simulink model "Waehrungsmodelle"  (R2014a)
settings: Solver=ode1  StartTime=0.0  StopTime=100  FixedStep=1  MaxStep=1  MinStep=1  RelTol=1e-3
(part 7 of 18)

== matlab function Waehrungsmodelle/Vollgeld Währungssystem/Banken/MATLAB Function ==
  data: EinlagenAenderungHaushalte input; KreditbedarfHaushalte input; KreditbedarfUnternehmen input; KreditbedarfHaushalteAusland input; KreditbedarfUnternehmenAusland input; KreditbedarfStaat input; Steuersatz input; Leitzins input; Mindestreservesatz input; MaximaleNotenbankGeldmenge input; KontoHaushalteOut output; KrediteHaushalteOut output; KrediteUnternehmenOut output; KrediteStaatOut output; KreditvergabeHaushalte output; KreditvergabeUnternehmen output; KreditvergabeStaat output; KreditrueckzahlungHaushalte output; KreditrueckzahlungUnternehmen output; KreditrueckzahlungStaat output; BankgewinnNachSteuern output; BankenSteuern output; BankKontostand output; Bankenzinssatz output; KrediteUnternehmenAuslandOut output; KreditrueckzahlungUnternehmenAusland output; KreditvergabeUnternehmenAusland output; KrediteHaushalteAuslandOut output; KreditrueckzahlungHaushalteAusland output; KreditvergabeHaushalteAusland output
function [KontoHaushalteOut, KrediteHaushalteOut, KrediteUnternehmenOut, KrediteStaatOut, ... 
            KreditvergabeHaushalte, KreditvergabeUnternehmen, KreditvergabeStaat, ...
            KreditrueckzahlungHaushalte, KreditrueckzahlungUnternehmen, KreditrueckzahlungStaat, ...
            BankgewinnNachSteuern, BankenSteuern, BankKontostand, Bankenzinssatz, ...
            KrediteUnternehmenAuslandOut, KreditrueckzahlungUnternehmenAusland, KreditvergabeUnternehmenAusland, ...
            KrediteHaushalteAuslandOut, KreditrueckzahlungHaushalteAusland, KreditvergabeHaushalteAusland] = ...
    Banken(EinlagenAenderungHaushalte, KreditbedarfHaushalte, KreditbedarfUnternehmen, ...
            KreditbedarfHaushalteAusland, KreditbedarfUnternehmenAusland, KreditbedarfStaat, ...
            Steuersatz, Leitzins, Mindestreservesatz, MaximaleNotenbankGeldmenge)
% Submodell Banken zur Berechnung der Geld-Prozesse zwischen 
% Banken und Haushalten

% ANMERKUNG:
% Warum gibt es auf der einen Seite Kredite und Guthaben der Haushalte?
% Der überwigende Teil der Geldes MUSS den Haushalten gehören, da diese
% die Unternehmen und Banken besitzen. Ich vermute, dass es in einen
% demokratischen Staat nicht möglich ist, dass der Staat mehr Geld als 
% die Bevölkerung besitzt.
% Die ungleiche Geldverteilung ist dafür verantwortlich, dass die Haushalte
% auf der einen Seite Spareinlagen und Kredite haben. Ohne Spareinlagen wäre
% es aktuell nicht möglich Kredite überhaupt zu vergeben.

% Der Zinsspread ist die Prozentuale-Differenz der Zinsweitergabe bei
% Krediten und Anlagen
persistent Zinsspread;

% interner Zinssatz
persistent InternerZinssatz;

% aktuelle Kredithöhe der Unternehmen
persistent KrediteUnternehmen;

% aktuelle Kredithöhe des Staats
persistent KrediteStaat;

% aktuelle Kredithöhe der Haushalte
persistent KrediteHaushalte;

% aktuelle Kredithöhe der Unternehmen im Ausland
persistent KrediteUnternehmenAusland;

% aktuelle Kredithöhe der Haushalte im Ausland
persistent KrediteHaushalteAusland;

% aktueller Kontostand der Haushalte
persistent KontoHaushalte;

% Rückzahlungsdauer des Kredits
persistent Kreditrueckzahlungsdauer;

% Vermnögen der Bank aus den Gewinnen
persistent KontoBank;

    % Zinsspread 1%
    if isempty(Zinsspread)
       Zinsspread = 0.01;
    end 
    
    % interner Zinssatz auf den Leitzins festlegen
    if isempty(InternerZinssatz)
       InternerZinssatz = Leitzins;
    end     
    
    % Rückzahlungsdauer 15 Zeiteinheiten
    if isempty(Kreditrueckzahlungsdauer)
       Kreditrueckzahlungsdauer = 15;
    end     
   
    if isempty(KontoBank)
       KontoBank = 400;
    end   
    if isempty(KontoHaushalte)
       KontoHaushalte = 0;
    end   
    if isempty(KrediteHaushalte)
       KrediteHaushalte = 200;
    end     
    if isempty(KrediteUnternehmen)
       KrediteUnternehmen = 200;
    end 
    if isempty(KrediteStaat)
       KrediteStaat = 200;
    end     
    if isempty(KrediteUnternehmenAusland)
       KrediteUnternehmenAusland = 200;
    end     
    if isempty(KrediteHaushalteAusland)
       KrediteHaushalteAusland = 200;
    end   
    
    % Zinsspread an das Guthaben der Bank anpassen
    if KontoBank < 0
        Zinsspread = Zinsspread + 0.01;
    elseif KontoBank > 1000
        Zinsspread = max(Zinsspread - 0.01, 0.01);
    end
    
    % Habenzinsen berechnen
    HabenZinsen = KontoHaushalte * (InternerZinssatz - Zinsspread);
    KontoHaushalte = KontoHaushalte + HabenZinsen;
    
    % Ein- / Auszahlung
    KontoHaushalte = KontoHaushalte + EinlagenAenderungHaushalte;    
      
    % Maximale Kreditvergabe anhand des Mindestreservesatzes und der 
    % Spareinlagen der Haushalte
    MaximaleKreditvergabe = KontoHaushalte * (1 / Mindestreservesatz); 

    % Maximale Geldmenge, welche von der Notenbank zur Verfügung gestellt wird
    % Prüfung anhand der Maximalen Kreditvergabe, da Guthaben = Kredit    
    MaximaleKreditvergabe = max(MaximaleNotenbankGeldmenge, MaximaleKreditvergabe);
    
    Gesamtkredit = KrediteHaushalte + KrediteUnternehmen + KrediteStaat;
    MaximaleKreditvergabe = MaximaleKreditvergabe - Gesamtkredit;

    % Wenn genug Geld auf dem Konto ist, so wird ein prozenualer Anteil mit
    % dem neuen Kreditbedarf verrechnet ==> 10 %    
    if KontoHaushalte > KreditbedarfHaushalte && KreditbedarfHaushalte > 0
       AusgleichbarerGeldBedarf = KreditbedarfHaushalte * 0.1;
       KontoHaushalte = KontoHaushalte - AusgleichbarerGeldBedarf;
       KreditbedarfHaushalte = KreditbedarfHaushalte - AusgleichbarerGeldBedarf;
    end         

    % Kreditberechnung für Haushalte      
    [KrediteHaushalte, KreditvergabeHaushalte, KreditrueckzahlungHaushalte, ...
                        SollZinsenHaushalte, MaximaleKreditvergabe] = ...
        Kreditberechnung(KrediteHaushalte, KreditbedarfHaushalte, MaximaleKreditvergabe, ...
                        InternerZinssatz, Zinsspread, Kreditrueckzahlungsdauer);                    
    
    % Kreditberechnung für Staat   
    [KrediteStaat, KreditvergabeStaat, KreditrueckzahlungStaat, SollZinsenStaat, ...
                        MaximaleKreditvergabe] = ...
        Kreditberechnung(KrediteStaat, KreditbedarfStaat, MaximaleKreditvergabe, ...
                        InternerZinssatz, Zinsspread, Kreditrueckzahlungsdauer);                    

    % Kreditberechnung für Unternehmen   
    [KrediteUnternehmen, KreditvergabeUnternehmen, KreditrueckzahlungUnternehmen, ...
                        SollZinsenUnternehmen, MaximaleKreditvergabe] = ...
        Kreditberechnung(KrediteUnternehmen, KreditbedarfUnternehmen, MaximaleKreditvergabe, ...
                        InternerZinssatz, Zinsspread, Kreditrueckzahlungsdauer);

    % Kreditberechnung für Haushalte im Ausland
    [KrediteHaushalteAusland, KreditvergabeHaushalteAusland, KreditrueckzahlungHaushalteAusland, ...
                        SollZinsenHaushalteAusland, MaximaleKreditvergabe] = ...
        Kreditberechnung(KrediteHaushalteAusland, KreditbedarfHaushalteAusland, MaximaleKreditvergabe, ...
                        InternerZinssatz, Zinsspread, Kreditrueckzahlungsdauer);                                        

    % Kreditberechnung für Unternehmen im Ausland
    [KrediteUnternehmenAusland, KreditvergabeUnternehmenAusland, KreditrueckzahlungUnternehmenAusland, ...
                        SollZinsenUnternehmenAusland, MaximaleKreditvergabe] = ...
        Kreditberechnung(KrediteUnternehmenAusland, KreditbedarfUnternehmenAusland, MaximaleKreditvergabe, ...
                        InternerZinssatz, Zinsspread, Kreditrueckzahlungsdauer);                    
                    
    % Berechnung der Notenbankkredite
    NotenbankKredite = (KrediteHaushalte + KrediteUnternehmen + KrediteStaat + ...
                    KrediteHaushalteAusland + KrediteUnternehmenAusland) - (KontoBank + KontoHaushalte);
    NotenbankKredite = max(NotenbankKredite, 0);
    NotenbankZinsen = NotenbankKredite * Leitzins;
    KontoBank = KontoBank - NotenbankZinsen;   
    
    % Gewinnberechnung der Bank
    SollZinsen = SollZinsenHaushalte + SollZinsenStaat + SollZinsenUnternehmen ...
                + SollZinsenHaushalteAusland + SollZinsenUnternehmenAusland;
    Bankgewinn = SollZinsen - HabenZinsen;
    
    % Steuerberechnung der Bank
    BankenSteuern = max(Bankgewinn * Steuersatz, 0);
    BankgewinnNachSteuern = Bankgewinn - BankenSteuern;
    
    % Kontostand der Bank berechnen
    KontoBank = KontoBank + Bankgewinn - BankenSteuern;
    
    % Zinssätze anpassen (Zinsänderung anpassen y = -0.00005x + 0.0025;
    Zinsaenderung = -0.00005 * BankgewinnNachSteuern + 0.001;
    Zinsaenderung = min(0.01, max(Zinsaenderung, -0.01));
    InternerZinssatz = InternerZinssatz + Zinsaenderung;
    
    if InternerZinssatz > 1
       InternerZinssatz = 0.1; 
    end
    
    KrediteStaatOut = KrediteStaat;
    KrediteUnternehmenOut = KrediteUnternehmen;
    KrediteHaushalteOut = KrediteHaushalte;
    KrediteUnternehmenAuslandOut = KrediteUnternehmenAusland;
    KrediteHaushalteAuslandOut = KrediteHaushalteAusland;    
    KontoHaushalteOut = KontoHaushalte;    
    BankKontostand = KontoBank;
    Bankenzinssatz = InternerZinssatz;

== matlab function Waehrungsmodelle/Währungssystem3/Umwelt/Umwelt ==
  data: Ressourcenbedarf input; AbgebauteRessourcen output; VorhandeneRessourcenOut output; Umweltqualitaet output
function [AbgebauteRessourcen, VorhandeneRessourcenOut, Umweltqualitaet] = Umwelt(Ressourcenbedarf)
%# Submodell zum Prozessablauf der Umwelt und der Ressourcen


% Vorhandene Ressourcen
persistent VorhandeneRessourcen;

% Initiale Ressourcen
InitialeRessourcen = 2500;
% Maximale Abbaurate
MaximaleAbbaurate = 0.1;
% Ressourcenregenerationsrate
Ressourcenregenerationsrate = 0.02;
    
% Vorhandene Ressourcen Initial
if isempty(VorhandeneRessourcen)
   VorhandeneRessourcen = InitialeRessourcen;
end

    % Berechnung der maximal abbaubaren Ressourcen
    MaximalAbbaubareRessourcen = VorhandeneRessourcen * MaximaleAbbaurate;
    
    % abgebaute Ressourcen
    AbgebauteRessourcen = min(MaximalAbbaubareRessourcen, Ressourcenbedarf);       
    VorhandeneRessourcen = VorhandeneRessourcen - AbgebauteRessourcen;
    
    % Ressourcen Regeneration
    VorhandeneRessourcen = VorhandeneRessourcen * (1  + Ressourcenregenerationsrate);    
    
    % Umweltqualitaet berechnen
    Umweltqualitaet = max(min(VorhandeneRessourcen / InitialeRessourcen, 1), 0);
        
    VorhandeneRessourcenOut = VorhandeneRessourcen;

== matlab function Waehrungsmodelle/Währungssystem3/Wechselkursberechnung/MATLAB Function ==
  data: GueterpreisAuslandInEigenwaehrung output; GueterpreisAusland input; Wechselkursfaktor output; GueterKonsumImInlandVomAusland input; GueterKonsumImAuslandVomInland input; GesamterGueterKonsumImAuslandVomInlandOut output; GesamterGueterKonsumImInlandVomAuslandOut output
function [GueterpreisAuslandInEigenwaehrung, Wechselkursfaktor, GesamterGueterKonsumImAuslandVomInlandOut, GesamterGueterKonsumImInlandVomAuslandOut] ...
        = Wechselkursberechnung(GueterpreisAusland, GueterKonsumImInlandVomAusland, GueterKonsumImAuslandVomInland)
%# Untermodul zur Berechnung eines realen Wechselkurses


% Aufsummierter Güterkonsum vom Ausland mit produzierten Gütern aus dem Inland
persistent GesamterGueterKonsumImAuslandVomInland;          
        
% Aufsummierter Güterkonsum vom Inland mit produzierten Gütern aus dem Ausland
persistent GesamterGueterKonsumImInlandVomAusland;    

% GesamterGueterKonsumImAuslandVomInland Initial
if isempty(GesamterGueterKonsumImAuslandVomInland)
   GesamterGueterKonsumImAuslandVomInland = 1;
end

% GueterKonsumImInlandVomAusland Initial
if isempty(GesamterGueterKonsumImInlandVomAusland)
   GesamterGueterKonsumImInlandVomAusland = 1;
end

GesamterGueterKonsumImAuslandVomInland = GesamterGueterKonsumImAuslandVomInland + GueterKonsumImAuslandVomInland;
GesamterGueterKonsumImInlandVomAusland = GesamterGueterKonsumImInlandVomAusland + GueterKonsumImInlandVomAusland;
   
% Berechnung eines realen Wechselkurses
Wechselkursfaktor =  GesamterGueterKonsumImInlandVomAusland / GesamterGueterKonsumImAuslandVomInland;

% Güterpreis der importierten Waren in Inländischer Währung
GueterpreisAuslandInEigenwaehrung = GueterpreisAusland * Wechselkursfaktor;

% Zustandswerte ausgeben
GesamterGueterKonsumImAuslandVomInlandOut = GesamterGueterKonsumImAuslandVomInland;
GesamterGueterKonsumImInlandVomAuslandOut = GesamterGueterKonsumImInlandVomAusland;

== matlab function Waehrungsmodelle/Gedecktes Währungssystem/Deckungsmaterialschöpfung/MATLAB Function ==
  data: NachfrageDeckungsmaterial input; RessourcenMengeDeckungsmaterial output; PreisDeckungsmaterialOut output; AngebotsMengeDeckungsmaterial output; Ressourcenabbaumenge output
function [RessourcenMengeDeckungsmaterial, PreisDeckungsmaterialOut, AngebotsMengeDeckungsmaterial, Ressourcenabbaumenge] = ...
    SchoepfungDeckungsmaterial(NachfrageDeckungsmaterial)
%# Submodul zur Berechnung der Notenbankprozesse

% Abbauzyklen
persistent Abbauzyklus;

% abgebauter Vorrat an dem Deckungsmaterial
persistent VorratDeckungsmaterial;

% Preis des Deckungsmaterial
persistent PreisDeckungsmaterial;

    % Anfänglicher Preis für das Deckungsmaterial
    InitPreisDeckungsmaterial = 10;

    if isempty(VorratDeckungsmaterial)
       VorratDeckungsmaterial = 100;
    end  
    if isempty(Abbauzyklus)
       Abbauzyklus = 1;
    end  
    if isempty(PreisDeckungsmaterial)
       PreisDeckungsmaterial = InitPreisDeckungsmaterial;
    end  
        
    Abbauzyklus = Abbauzyklus + 1;
        
    % Abbaumenge pro Zeiteinheit
    Ressourcenabbaumenge = 70 - 20 * (Abbauzyklus ^ 0.2);    
    VorratDeckungsmaterial = VorratDeckungsmaterial + Ressourcenabbaumenge;
    
    if VorratDeckungsmaterial < NachfrageDeckungsmaterial * 3
        PreisAenderungsfaktor = max(1, NachfrageDeckungsmaterial / Ressourcenabbaumenge);
    elseif VorratDeckungsmaterial > NachfrageDeckungsmaterial * 25
        PreisAenderungsfaktor = min(1, max(0.9, NachfrageDeckungsmaterial / Ressourcenabbaumenge));
    else
        PreisAenderungsfaktor =  min(1.2, NachfrageDeckungsmaterial / Ressourcenabbaumenge);
    end
    
    PreisDeckungsmaterial = PreisDeckungsmaterial * (2+PreisAenderungsfaktor) / 3;
    
    % Auf Grund der Deckung ist der Preis für das Deckungsmaterial niemals
    % unter dem ursprünglichen Geld. Auf Grund des Angebots und der
    % Nachfrage ist es dennoch möglich, dass der Preis schwankt
    if PreisDeckungsmaterial < InitPreisDeckungsmaterial
        PreisDeckungsmaterial = InitPreisDeckungsmaterial;
    end
    
    if VorratDeckungsmaterial > NachfrageDeckungsmaterial
        AngebotsMengeDeckungsmaterial = NachfrageDeckungsmaterial;
        
    else
        AngebotsMengeDeckungsmaterial = VorratDeckungsmaterial;
    end
    
    VorratDeckungsmaterial = VorratDeckungsmaterial - AngebotsMengeDeckungsmaterial;           
    RessourcenMengeDeckungsmaterial = VorratDeckungsmaterial;
    PreisDeckungsmaterialOut = PreisDeckungsmaterial;

== matlab function Waehrungsmodelle/Gedecktes Währungssystem/Umwelt/Umwelt ==
  data: Ressourcenbedarf input; AbgebauteRessourcen output; VorhandeneRessourcenOut output; Umweltqualitaet output
function [AbgebauteRessourcen, VorhandeneRessourcenOut, Umweltqualitaet] = Umwelt(Ressourcenbedarf)
%# Submodell zum Prozessablauf der Umwelt und der Ressourcen


% Vorhandene Ressourcen
persistent VorhandeneRessourcen;

% Initiale Ressourcen
InitialeRessourcen = 2500;
% Maximale Abbaurate
MaximaleAbbaurate = 0.1;
% Ressourcenregenerationsrate
Ressourcenregenerationsrate = 0.02;
    
% Vorhandene Ressourcen Initial
if isempty(VorhandeneRessourcen)
   VorhandeneRessourcen = InitialeRessourcen;
end

    % Berechnung der maximal abbaubaren Ressourcen
    MaximalAbbaubareRessourcen = VorhandeneRessourcen * MaximaleAbbaurate;
    
    % abgebaute Ressourcen
    AbgebauteRessourcen = min(MaximalAbbaubareRessourcen, Ressourcenbedarf);       
    VorhandeneRessourcen = VorhandeneRessourcen - AbgebauteRessourcen;
    
    % Ressourcen Regeneration
    VorhandeneRessourcen = VorhandeneRessourcen * (1  + Ressourcenregenerationsrate);    
    
    % Umweltqualitaet berechnen
    Umweltqualitaet = max(min(VorhandeneRessourcen / InitialeRessourcen, 1), 0);
        
    VorhandeneRessourcenOut = VorhandeneRessourcen;

== matlab function Waehrungsmodelle/Gedecktes Währungssystem/Unternehmen/MATLAB Function ==
  data: Inflation output; Rohstoffbedarf output; ArbeitsplaetzeUnternehmen output; GueterangebotInland output; ArbeitslohnOut output; Erwerbsfaehige input; BenoetigterArbeitsbedarfUnternehmen output; GueterpreisOut output; NeueKreditvergabeUnternehmen input; KreditrueckzahlungUnternehmen input; SteuernUnternehmen output; RessourcenAbgabeSteuer output; KreditbedarfInland output; Rohstoffe input; GueterkonsumInland input; GueterkonsumAusland input; RessourcenAbgabeSteuersatz input; KreditZinssatzInland input; KreditZinssatzAusland input; Steuersatz input; KreditbedarfAusland output; TechnischeVerbesserungRationalitaetOut output; TechnischeVerbesserungRessourcenOut output; Wirtschaftswachstum output; GueterangebotAusland output; NeueKreditvergabeUnternehmenAusland input; KreditrueckzahlungUnternehmenAusland input
function [Inflation, Rohstoffbedarf, ArbeitsplaetzeUnternehmen, GueterangebotInland, ...
            ArbeitslohnOut, BenoetigterArbeitsbedarfUnternehmen, GueterpreisOut, ...
            SteuernUnternehmen, RessourcenAbgabeSteuer, KreditbedarfInland, KreditbedarfAusland,  ...
            TechnischeVerbesserungRationalitaetOut, TechnischeVerbesserungRessourcenOut, ...
            Wirtschaftswachstum, GueterangebotAusland] = ...
   Unternehmen(Erwerbsfaehige, NeueKreditvergabeUnternehmen, KreditrueckzahlungUnternehmen, ...
            Rohstoffe, GueterkonsumInland, GueterkonsumAusland, RessourcenAbgabeSteuersatz, ...
            KreditZinssatzInland, KreditZinssatzAusland, Steuersatz, ...
            NeueKreditvergabeUnternehmenAusland, KreditrueckzahlungUnternehmenAusland)
        %# Submodul zur Berechnung der Prozessabläufe in Beziehung mit den Unternehmen

% Arbeitslohn
persistent Arbeitslohn;          
        
% Geldbestand
persistent Geldbestand;  
        
% Rohstoffbestand
persistent Rohstoffbestand;   
        
% produzierter Güterbestand
persistent Gueterbestand;   

% Preis zu dem das produzierte Gut verkauft wird
persistent Gueterpreis;  

% technische Effizienzverbesserung bzgl. der Rationalisierung der Arbeiter
persistent TechnischeVerbesserungRationalitaet;   

% technische Effizienzverbesserung bzgl. der Ressourcenverwendung
persistent TechnischeVerbesserungRessourcen;

% Letzte Anzahl an Mitarbeitern
persistent LetzteArbeitsplaetzeUnternehmen;

% Umsatz / Einnahmen
persistent Einnahmen;

% alte Inflation
persistent InflationAlt;

% Geldbestand Initial
if isempty(Geldbestand)
   Geldbestand = 50;
end
% Arbeitslohn Initial
if isempty(Arbeitslohn)
   Arbeitslohn = 3.5;
end
% Rohstoffbestand Initial
if isempty(Rohstoffbestand)
   Rohstoffbestand = 50;
end
% Güterbestand Initial
if isempty(Gueterbestand)
   Gueterbestand = 50;
end 
% Güterpreis Initial
if isempty(Gueterpreis)
   Gueterpreis = 3;
end 
% technische Effizienzverbesserung Rationalisierung Initial
if isempty(TechnischeVerbesserungRessourcen)
   TechnischeVerbesserungRessourcen = 1;
end
% technische Effizienzverbesserung Ressourcenverwendung Initial
if isempty(TechnischeVerbesserungRationalitaet)
   TechnischeVerbesserungRationalitaet = 1;
end
% Umsatz / Einnahmen Initial
if isempty(Einnahmen)
   Einnahmen = 0;
end
if isempty(InflationAlt)
   InflationAlt = 0;
end
% Letzte Anzahl an Mitarbeitern
if isempty(LetzteArbeitsplaetzeUnternehmen)
   LetzteArbeitsplaetzeUnternehmen = 20;
end

% Steigerung der Effizienzen bei technischen Verbesserungen Rationalität
EffizienzsteigerungRationalitaet = 0.04;
% Steigerung der Effizienzen bei technischen Verbesserungen Ressourcen
EffizienzsteigerungRessourcen = 0.02;
% Kosten einer technischen Verbesserung
Verbesserungskosten = 20;
% Steigerung der Kosten bei technischen Verbesserungen
Verbesserungskostensteigerung = 0.2;
% Angestrebter Gewinn
AngestrebterGewinn = 0.1;
% Maximale Preissteierung
MaximalePreissteierung = 0.15;
% Speicherung des letzten Güterpreises
AlterGueterpreis = Gueterpreis;
% Speicherung der letzten Einnahmen
AlteEinnahmen = Einnahmen;
% Menge produzierter Güter pro Mitarbeiter
ProduzierteMengeProMitarbeiter = 1.2;
% Gehaltssteigerung bei Rationalisierung und Gewinn
Gehaltssteigerung = 0.05;
% angestrebter Gütervorrat
GewuenschterGuetervorrat = 200;
% angestrebter Geldbestand
GewuenschterGeldbestand = 200;
% Maximale Entlassungen in Prozent
MaximaleEntlassungsrate = 0.2;

    % vergebene Kredite
    Geldbestand = Geldbestand + NeueKreditvergabeUnternehmen + NeueKreditvergabeUnternehmenAusland;
    % Ratenzahlung der aktuelen Kredite
    Geldbestand = Geldbestand - KreditrueckzahlungUnternehmen + KreditrueckzahlungUnternehmenAusland;

    % Berechnung der Ressourcenangabe
    RessourcenAbgabeSteuer = max(0, RessourcenAbgabeSteuersatz) * Rohstoffe;
    Rohstoffbestand = Rohstoffbestand + Rohstoffe;
    
    % In- und Auslandskonsum summieren
    Gueterkonsum = GueterkonsumInland + GueterkonsumAusland;
    
    % Güterbestand nach den von abgenommene Güter der Haushalten bei 
    % der letzten Zeiteinheit 
    Gueterbestand = Gueterbestand - Gueterkonsum;
    
    % Berechnung der Einnahmen
    Einnahmen = Gueterkonsum * Gueterpreis;
    
    % Berechnung der zu produzierenden Gütermenge (mit 30% Reserve) wenn
    % der Bestand kleiner als 200% des Güterkonsums in einer Zeiteinheit
    % Dabei werden 50 Güter als Reserve in Bestand vorgehalten
    if Gueterbestand < Gueterkonsum * 2
        ProduzierndeGuetermenge = max(5, (1.3 * Gueterkonsum) - (Gueterbestand - GewuenschterGuetervorrat));  
    elseif Gueterbestand < GewuenschterGuetervorrat
        ProduzierndeGuetermenge = Gueterkonsum + (GewuenschterGuetervorrat - Gueterbestand);
    else
       ProduzierndeGuetermenge = max(5, Gueterkonsum / 2);      
    end
    
    % Produktiongüter pro Mitarbeiter in Abhängigkeit
    % der technischen Verbesserung (normal 2 Güter pro Mitarbeiter)
    ProduktionProMitarbeiter = (((1 + EffizienzsteigerungRationalitaet) ^ TechnischeVerbesserungRationalitaet) * ProduzierteMengeProMitarbeiter);
    
    % Ressourcen pro hergestelltes Gut in Abhängigkeit
    % der technischen Verbesserung (normal 1 Güter pro Ressource)    
    RessourcenProGut = (1 / (1 + EffizienzsteigerungRessourcen)) ^ TechnischeVerbesserungRessourcen;
    
    % Zur Berechnung der benötigten Arbeitskraft im nächsten Zeitabschnitt´
    BenoetigterArbeitsbedarfUnternehmen = floor(ProduzierndeGuetermenge / ProduktionProMitarbeiter) + 1;           
    
    % Berechnung der maximal erstellbaren Gütermenge
    MaximaleGueterherstellungErwerbstaetige = Erwerbsfaehige * ProduktionProMitarbeiter;
    MaximaleGueterherstellungRohstoffe = Rohstoffbestand / RessourcenProGut;    
    % Entweder ist die Herstellung durch die Nachfrage, den Arbeitskreaften
    % oder den Ressourcen beschränkt
    Gueterherstellung = min(ProduzierndeGuetermenge, min(MaximaleGueterherstellungErwerbstaetige, MaximaleGueterherstellungRohstoffe));
    Gueterherstellung = max(Gueterherstellung, 0);  
    
    % Berechnung der aktuellen Arbeitsplätze
    ArbeitsplaetzeUnternehmen = floor(Gueterherstellung / ProduktionProMitarbeiter)+1;
    
    % Berechnung der maximalen möglichen Entlassungen
    % Es können max. 20% der Mitarbeiter entlassen werden    
    if ArbeitsplaetzeUnternehmen < LetzteArbeitsplaetzeUnternehmen * (1-MaximaleEntlassungsrate)
        ArbeitsplaetzeUnternehmen = LetzteArbeitsplaetzeUnternehmen * (1-MaximaleEntlassungsrate);
        MaximaleGueterherstellungErwerbstaetige = ArbeitsplaetzeUnternehmen * ProduktionProMitarbeiter;
        Gueterherstellung = min(ProduzierndeGuetermenge, min(MaximaleGueterherstellungErwerbstaetige, MaximaleGueterherstellungRohstoffe));        
    end
    
    % Vergleich der Arbeitsnachfrage mit dem Arbeitsangebot
    ArbeitsangebotsNachfrageQuotient = ArbeitsplaetzeUnternehmen / Erwerbsfaehige;
    % Anpassung der Arbeitslöhne an das Angebot und die Nachfrage der
    % Arbeitsplaetze - max 3% Lohnsenkung oder Lohnsteigerung
    ArbeitsangebotsNachfrageQuotient= max(0.94,min(1.04,(ArbeitsangebotsNachfrageQuotient + 0.3)));
    Arbeitslohn = Arbeitslohn * ArbeitsangebotsNachfrageQuotient;
    
    % Berechnung der aktuell verbrauchten Ressourcen
    Rohstoffbestand = Rohstoffbestand - (floor(Gueterherstellung * RessourcenProGut)+1);
    
    % hergestellte Gütermenge
    Gueterbestand = Gueterbestand + Gueterherstellung;
    
    % Als Export-Angebot werden 30% der Güter vorgesehen
    GueterangebotAusland = Gueterbestand * 0.3;
    GueterangebotInland = Gueterbestand - GueterangebotAusland;          
    
    % Berechnung der Gehälter
    Gehaelter = ArbeitsplaetzeUnternehmen * Arbeitslohn;
    
    % Vorteil einer Investitionen-Rationalität berechnen
    InvestPruefungProduktionProMitarbeiter = (((1 + EffizienzsteigerungRationalitaet) ^ (TechnischeVerbesserungRationalitaet + 1)) * 2);
    InvestPruefungArbeitsplaetzeUnternehmen = floor(Gueterherstellung / InvestPruefungProduktionProMitarbeiter)+1;    
    InvesteinsparungRationalitaet = Arbeitslohn * (ArbeitsplaetzeUnternehmen - InvestPruefungArbeitsplaetzeUnternehmen);
    % Vorteil einer Investitionen-Ressourceneffizienz berechnen
    InvestPruefungRessourcenProGut = (1 / (1 + EffizienzsteigerungRessourcen)) ^ (TechnischeVerbesserungRessourcen + 1);
    InvestPruefungRessourcenbedarf = floor(Gueterherstellung * InvestPruefungRessourcenProGut)+1;    
    InvesteinsparungRessourcenbedarf = RessourcenAbgabeSteuersatz * ((Gueterherstellung * RessourcenProGut) - InvestPruefungRessourcenbedarf);    
    
    % Kosten für die nächste Investitionsstufe berechnen
    InvestkostenRationalitaet = Verbesserungskosten * (1 + Verbesserungskostensteigerung) ^ (TechnischeVerbesserungRationalitaet + 1);
    InvestkostenRessourcenEffizienz = Verbesserungskosten * (1 + Verbesserungskostensteigerung) ^ (TechnischeVerbesserungRessourcen + 1);
    
    % Prüfen, ob und welche Investition mehr Sinn macht
    % Das vorhandene Geld muss dabei doppelt so hoch sein, damit nicht mit
    % dem letzten Geld Investitionen durchgeführt werden
    Investition = 0;
    if (InvesteinsparungRationalitaet > InvesteinsparungRessourcenbedarf) && Geldbestand > InvestkostenRationalitaet*2 && InvesteinsparungRationalitaet > 0
        % Verbesserung Rationalität
        TechnischeVerbesserungRationalitaet = TechnischeVerbesserungRationalitaet + 1;
        Investition = InvestkostenRationalitaet;
        % Anstieg des Arbeitslohn auf Grund der Rationalitätsgewinne 
        Arbeitslohn = Arbeitslohn * (1 + Gehaltssteigerung);
    elseif Geldbestand > InvestkostenRessourcenEffizienz*2 && InvesteinsparungRessourcenbedarf > 0;
        % Verbesserung Ressourceneffizienz
        TechnischeVerbesserungRessourcen = TechnischeVerbesserungRessourcen + 1;
        Investition = InvestkostenRessourcenEffizienz;
    end
    
    % Ausgaben berechnen
    Ausgaben = RessourcenAbgabeSteuer + Gehaelter;
    
    % Der Preis der produzierten Warten richtet sich NICHT nach der Nachfrage 
    % und dem Angebot, sondern nach den Herrstellungskosten und dem 
    % angestrebten Gewinn. Welches ist der niedrigste Preis, damit das 
    % Unternehmen den angestrebten Gewinn erwirtschaftet und Investieren
    % kann
    Herstellkosten = Ausgaben / Gueterherstellung;
    % Es gibt eine maximale Preisteigerung welche durchgesetzt werden kann
    MaximalerGueterpreis = (1 + MaximalePreissteierung) * Gueterpreis;
    Gueterpreis = min(MaximalerGueterpreis, Herstellkosten * (1 + AngestrebterGewinn));   
    
    % Berechnung der Inflation
    Inflation = (InflationAlt + (Gueterpreis / AlterGueterpreis) - 1) / 2;
    InflationAlt = Inflation;
                
    % Gewinnberechnung
    Gewinn = Einnahmen - Ausgaben;            
    
    if Gewinn > 0
        % Anstieg des Arbeitslohn auf Grund der Gewinnsteigerung               
        Arbeitslohn = Arbeitslohn * (1 + Gehaltssteigerung);  
        
        % Steuerberechnung vom Gewinn
        SteuernUnternehmen = Gewinn * Steuersatz;
    else
        SteuernUnternehmen = 0;
    end

    Geldbestand = Geldbestand + Gewinn - (SteuernUnternehmen + Investition);
       
    % Wenn notwendig, neuen Kredit beantragen
    if Geldbestand < GewuenschterGeldbestand                
        % Kreditbedarf berechnen
        Kreditbedarf = GewuenschterGeldbestand - Geldbestand;
    else 
        Kreditbedarf = 0;
    end         
    
    % Kreditbedarf auf In- und Ausland aufteilen
    % Der Kredit mit dem geringeren Zinssatz wird bevorzugt und 70%
    % verwendet. Der teurere Kredit wird mit 30% verwendet.
    if KreditZinssatzInland <= KreditZinssatzAusland
        KreditbedarfInland = Kreditbedarf * 0.7;
        KreditbedarfAusland = Kreditbedarf * 0.3;
    else
        KreditbedarfAusland = Kreditbedarf * 0.7;
        KreditbedarfInland = Kreditbedarf * 0.3;        
    end

    % Berechnung der benötigten Ressourcen im nächsten Zeitabschnitt    
    Rohstoffbedarf = max(0, floor(Gueterherstellung * RessourcenProGut) + GewuenschterGuetervorrat - Rohstoffbestand);            
    
    % Auf Grund der Angebots-/Nachfragesituation kann der Güterpreis nicht
    % unter dem Arbeitslohn sein
    Gueterpreis = min(Gueterpreis, Arbeitslohn);
    % Wenn kein Konsum stattgefunden hat sinkt der Preis
    if GueterkonsumInland == 0
        Gueterpreis = Gueterpreis * (1-MaximalePreissteierung);
    end
    
    
    Wirtschaftswachstum = (Einnahmen / AlteEinnahmen) - 1;
    
    ArbeitslohnOut = Arbeitslohn;
    GueterpreisOut = Gueterpreis;
    TechnischeVerbesserungRationalitaetOut = TechnischeVerbesserungRationalitaet;
    TechnischeVerbesserungRessourcenOut = TechnischeVerbesserungRessourcen;
    LetzteArbeitsplaetzeUnternehmen = ArbeitsplaetzeUnternehmen;

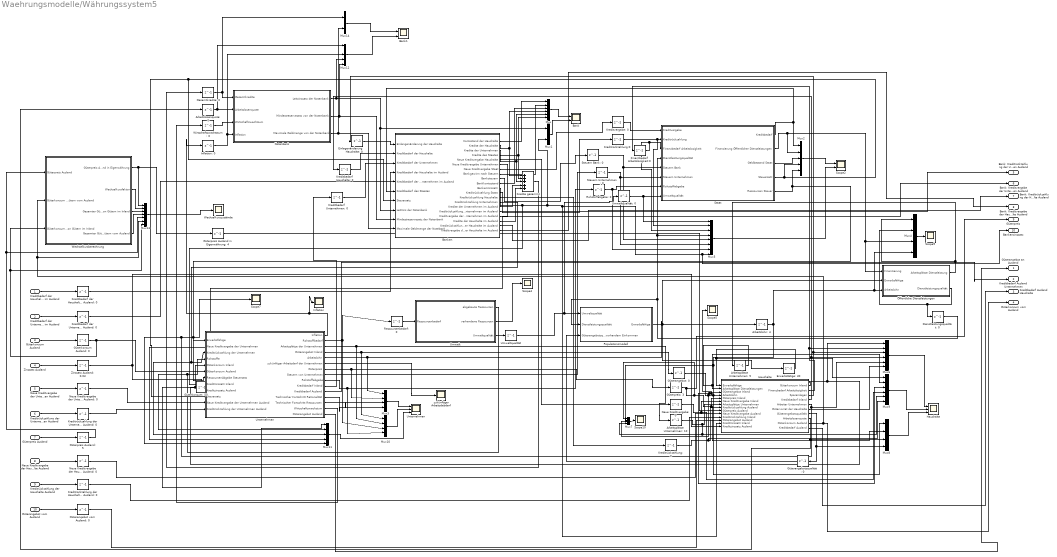
== system Waehrungsmodelle/Währungssystem5 ==
  Kreditbedarf der Haushalte im Ausland : Inport
  Kreditbedarf der Unternehmen im Ausland : Inport  Port=2
  Güterkonsum Ausland : Inport  Port=3
  Zinssatz Ausland : Inport  Port=4
  Neue Kreditvergabe der Unternehmen Ausland : Inport  Port=5
  Kreditrückzahlung der Unternehmen Ausland : Inport  Port=6
  Güterpreis Ausland : Inport  Port=7
  Neue Kreditvergabe der Haushalte Ausland : Inport  Port=8
  Kreditrückzahlung der Haushalte Ausland : Inport  Port=9
  Güterangebot vom  Ausland : Inport  Port=10
  Arbeitslohn: 4 : Delay  DelayLength=1  InitialCondition=4
  Arbeitslosenquote: 0 : Delay  DelayLength=1  InitialCondition=0
  "Arbeitsplätze Unternehmen: 10 " : Delay  DelayLength=1  InitialCondition=10
  Arbeitsplätze Unternehmen: 5 : Delay  DelayLength=1  InitialCondition=5
  Bank : Scope  NumInputPorts=2
      settings: ShowLegends=on  TimeRange=20  YMin=-500~0  YMax=500~0.1
  Bank1 : Scope  NumInputPorts=2
      settings: ShowLegends=on  TimeRange=20  YMin=-500~-0.5  YMax=10000~0.5  SaveName=ScopeData3
  Banken : Subsystem
  Dienstleistungsqualität: 0 : Delay  DelayLength=1  InitialCondition=0
  Einlagenänderung Haushalte: 0 : Delay  DelayLength=1  InitialCondition=0
  Erwerbstätige: 30 : Delay  DelayLength=1  InitialCondition=30
  Finanzbedarf Arbeitslosigkeit:0 : Delay  DelayLength=1  InitialCondition=0
  Gesamtkredite: 0 : Delay  DelayLength=1  InitialCondition=0
  Güterangebot vom  Ausland: 0 : Delay  DelayLength=1  InitialCondition=0
  Güterangebot: 0 : Delay  DelayLength=1  InitialCondition=0
  Güterangebotsqualität: 0 : Delay  DelayLength=1  InitialCondition=0
  Güterkonsum Ausland: 0 : Delay  DelayLength=1  InitialCondition=0
  Güterkonsum: 50 : Delay  DelayLength=1  InitialCondition=50
  Güterpreis Ausland in Eigenwährung: 4 : Delay  DelayLength=1  InitialCondition=4
  Güterpreis Ausland: 5 : Delay  DelayLength=1  InitialCondition=5
  Güterpreis: 3 : Delay  DelayLength=1  InitialCondition=3
  Haushalte : Subsystem
  "Haushalte " : Scope  NumInputPorts=3
      settings: TickLabels=on  ShowLegends=on  TimeRange=100  YMin=-50~0~0  YMax=150~100~1
  Inflation : Scope
      settings: ShowLegends=on  TimeRange=100  YMin=-0.1  YMax=0.15  SaveName=ScopeData12
  Inflation: 0 : Delay  DelayLength=1  InitialCondition=0
  Kreditbedarf Haushalte: 0 : Delay  DelayLength=1  InitialCondition=0
  Kreditbedarf Unternehmen: 0 : Delay  DelayLength=1  InitialCondition=0
  Kreditbedarf der Haushalte im Ausland: 0 : Delay  DelayLength=1  InitialCondition=0
  Kreditbedarf der Unternehmen im Ausland: 0 : Delay  DelayLength=1  InitialCondition=0
  Kredite gesammt : Sum  Inputs=+++++
  Kreditrückzahlung der Haushalte Ausland: 0 : Delay  DelayLength=1  InitialCondition=0
  Kreditrückzahlung der Unternehmen Ausland: 0 : Delay  DelayLength=1  InitialCondition=0
  Kreditrückzahlung: 0 : Delay  DelayLength=1  InitialCondition=0
  Kreditrückzahlung:0 : Delay  DelayLength=1  InitialCondition=0
  Kreditvergabe: 0 : Delay  DelayLength=1  InitialCondition=0
  Mux : Mux  Inputs=6
  Mux1 : Mux  Inputs=2
  Mux{3..4,7..8,10} (5 alike) : Mux
  Mux11 : Mux  Inputs=5
  Mux12 : Mux  Inputs=5
  Mux13 : Mux  Inputs=7
  Mux14 : Mux  Inputs=2
  Mux2 : Mux  Inputs=5
  Mux5 : Mux  Inputs=8
  Mux6 : Mux  Inputs=6
  Mux9 : Mux  Inputs=6
  Neue Kreditvergabe der Haushalte Ausland: 0 : Delay  DelayLength=1  InitialCondition=0
  Neue Kreditvergabe der Unternehmen Ausland: 0 : Delay  DelayLength=1  InitialCondition=0
  Neue Kreditvergabe: 0 : Delay  DelayLength=1  InitialCondition=0
  Notenbank : Subsystem
  Populationsmodell : Subsystem
  Ressourcenbedarf: 0 : Delay  DelayLength=1  InitialCondition=0
  Rohstoffabgabe: 0 : Delay  DelayLength=1  InitialCondition=0
  Scope{4..5,7,9..10} (5 alike) : Scope
      Scope10 settings: ShowLegends=on  TimeRange=100  YMin=0  YMax=120  SaveName=ScopeData10
      Scope4 settings: SaveName=ScopeData4
      Scope5 settings: TimeRange=10  YMin=0  YMax=10  SaveName=ScopeData5
      Scope7 settings: ShowLegends=on  TimeRange=10  YMin=9  YMax=15  SaveName=ScopeData7
      Scope9 settings: TickLabels=on  ShowLegends=on  TimeRange=100  YMin=0  YMax=40  SaveName=ScopeData9
  Scope2 : Scope  NumInputPorts=2
      settings: ShowLegends=on  TimeRange=100  YMin=-100~0  YMax=300~500  SaveName=ScopeData2
  Staat : Subsystem
  Steuern Bank: 0 : Delay  DelayLength=1  InitialCondition=0
  Steuern Unternehmen: 0 : Delay  DelayLength=1  InitialCondition=0
  Umwelt : Subsystem
  Umweltqualität : Delay  DelayLength=1  InitialCondition=0
  Umweltqualität: 0 : Delay  DelayLength=1  InitialCondition=0
  Unternehmen : Subsystem
  "Unternehmen " : Scope  NumInputPorts=3
      settings: TickLabels=on  ShowLegends=on  TimeRange=100  YMin=2~-5~-5  YMax=50~200~100  SaveName=ScopeData6
  Wechselkursberechnung : Subsystem
  Wechselkurszustände : Scope
      settings: ShowLegends=on  TimeRange=100  YMin=0  YMax=1  SaveName=ScopeData11
  Wirtschaftswachtstum: 0 : Delay  DelayLength=1  InitialCondition=0
  Zinssatz Ausland: 0.03 : Delay  DelayLength=1  InitialCondition=0.03
  zukünftiger Arbeitsdebdarf : Scope
      settings: ShowLegends=on  TimeRange=10  YMin=9  YMax=15  SaveName=ScopeData14
  Öffentliche Dienstleistungen : Subsystem
  Güterangebot an  Ausland : Outport
  Kreditbedarf Ausland Unternehmen : Outport  Port=2
  Kreditbedarf Ausland Haushalte : Outport  Port=3
  Güterkonsum vom Ausland : Outport  Port=4
  Bank: Kreditrückzahlung der Unternemen Ausland : Outport  Port=5
  "Bank: Kreditvergabe der Unternemen Ausland " : Outport  Port=6
  Bank: Kreditrückzahlung der Haushalte Ausland : Outport  Port=7
  "Bank: Kreditvergabe der Haushalte Ausland " : Outport  Port=8
  Güterpreis : Outport  Port=9
  Bankenzinssatz : Outport  Port=10
  wires:
  Öffentliche Dienstleistungen/1(Arbeitsplätze Dienstleistung) -> Arbeitsplätze Unternehmen: 5/1, Mux4/1
  Staat/4(Steuersatz) -> Mux2/4, Banken/7(Steuersatz), Unternehmen/10(Steuersatz)
  Umwelt/3(Umweltqualität) -> Umweltqualität/1
  Staat/5(Ressourcen Steuer) -> Unternehmen/7(RessourcenAbgabe Steuersatz), Mux2/5
  Populationsmodell/1(Erwerbsfähige) -> Erwerbstätige: 30/1, Öffentliche Dienstleistungen/2(Erwerbsfähige)
  Unternehmen/7(Güterpreis) -> Mux3/2, Güterpreis: 3/1
  Unternehmen/5(Arbeitslohn) -> Mux3/1, Arbeitslohn: 4/1
  Unternehmen/4(Güterangebot Inland) -> Mux10/1, Güterangebot: 0/1
  Unternehmen/3(Arbeitsplätze der Unternehmen) -> Mux10/2, "Arbeitsplätze Unternehmen: 10 "/1
  Umwelt/1(abgebaute Ressourcen) -> Unternehmen/4(Rohstoffe), Mux11/2
  Haushalte/1(Güterkonsum Inland) -> Mux6/1, Güterkonsum: 50/1
  Haushalte/7(Güterangebotsqualität) -> Mux8/4, Güterangebotsqualität: 0/1
  Staat/2(Finanzierung Öffentlicher Dienstleistungen) -> Mux2/2, Öffentliche Dienstleistungen/1(Finanzierung), Mux4/3
  Haushalte/5(Arbeiter Unternehmen) -> Mux6/5, Scope7/1, Unternehmen/1(Erwerbsfähige), Mux11/5
  Haushalte/2(Finanzbedarf Arbeitslosigkeit) -> Finanzbedarf Arbeitslosigkeit:0/1, Mux6/2
  Unternehmen/8(Steuern von Unternehmen) -> Steuern Unternehmen: 0/1
  Unternehmen/9(Rohstoffabgabe) -> Mux10/4, Rohstoffabgabe: 0/1
  Haushalte/8(Arbeitslosenquote) -> Arbeitslosenquote: 0/1, Mux8/3
  Unternehmen/1(Inflation) -> Inflation/1, Inflation: 0/1
  Unternehmen/14(Wirtschaftswachstum) -> Wirtschaftswachtstum: 0/1
  Notenbank/1(Leitzinssatz der Notenbank) -> Mux12/4, Mux1/1, Banken/8(Leitzins der Notenbank)
  Notenbank/2(Mindestreservesatz von der Notenbank) -> Mux12/5, Banken/9(Mindestreservesatz der Notenbank)
  Notenbank/3(Maximale Geldmenge von der Notenbank) -> Banken/10(Maximale Geldmenge der Notebank), Mux14/2
  Banken/2(Kredite der Haushalte) -> Mux/4, Kredite gesammt/1
  Banken/3(Kredite der Unternehmen) -> Mux/6, Kredite gesammt/2
  Banken/4(Kredite des Staates) -> Mux/5, Kredite gesammt/3
  Banken/9(Banksteuern) -> Steuern Bank: 0/1
  Banken/7(Neue Kreditvergabe Staat) -> Kreditvergabe: 0/1
  Banken/12(Kreditrückzahlung Staat) -> Kreditrückzahlung:0/1
  Banken/13(Kreditrückzahlung Haushalte) -> Kreditrückzahlung: 0/1
  Banken/5(Neue Kreditvergabe Haushalte) -> Neue Kreditvergabe: 0/1
  Haushalte/3(Spareinlagen) -> Einlagenänderung Haushalte: 0/1, Mux6/3
  Haushalte/4(Kreditbedarf Inland) -> Kreditbedarf Haushalte: 0/1, Mux6/4
  Unternehmen/10(Kreditbedarf Inland) -> Kreditbedarf Unternehmen: 0/1
  Staat/1(Kreditbedarf) -> Banken/6(Kreditbedarf des Staates), Mux2/1
  Banken/6(Neue Kreditvergabe Unternehmen) -> Mux11/4, Unternehmen/2(Neue Kreditvergabe der Unternehmen)
  Banken/14(Kreditrückzahlung Unternehmen) -> Unternehmen/3(Kreditrückzahlung der Unternehmen), Mux11/3
  Banken/1(Kontostand der Haushalte) -> Mux/1
  Banken/8(Bankgewinn nach Steuern) -> Mux/2
  Banken/10(Bankkontostand) -> Mux/3
  Banken/11(Bankenzinssatz) -> Haushalte/13(Kreditzinssatz Inland), Bankenzinssatz/1, Mux5/8, Mux1/2, Unternehmen/8(Kreditzinssatz Inland)
  Unternehmen/13(Technischer Fortschritt Ressourcen) -> Mux3/3
  Unternehmen/12(Technischer Fortschritt Rationalität) -> Mux3/4
  Umwelt/2(verhandene Ressourcen) -> Scope4/1
  Kredite gesammt/1 -> Gesamtkredite: 0/1
  Gesamtkredite: 0/1 -> Notenbank/1(Gesamtkredite), Mux14/1
  Wirtschaftswachtstum: 0/1 -> Notenbank/3(Wirtschaftswachtsum)
  Inflation: 0/1 -> Mux12/3, Notenbank/4(Inflation)
  Ressourcenbedarf: 0/1 -> Umwelt/1(Ressourcenbedarf)
  Unternehmen/2(Rohstoffbedarf) -> Ressourcenbedarf: 0/1, Mux10/3
  Umweltqualität: 0/1 -> Mux5/1, Staat/8(Umweltqualität)
  Rohstoffabgabe: 0/1 -> Mux5/7, Staat/7(Rohstoffabgabe)
  Dienstleistungsqualität: 0/1 -> Populationsmodell/2(Dienstleistungsqualität), Staat/4(Dienstleistungsqualität), Mux5/4
  Steuern Unternehmen: 0/1 -> Mux5/6, Staat/6(Steuern Unternehmen)
  Steuern Bank: 0/1 -> Staat/5(Steuern Bank), Mux5/5
  Finanzbedarf Arbeitslosigkeit:0/1 -> Mux5/3, Staat/3(Finanzbedarf Arbeitslosigkeit)
  Kreditrückzahlung:0/1 -> Staat/2(Kreditrückzahlung), Mux5/2
  Kreditvergabe: 0/1 -> Staat/1(Kreditvergabe)
  Umweltqualität/1 -> Umweltqualität: 0/1, Populationsmodell/1(Umweltqualität)
  Öffentliche Dienstleistungen/2(Dienstleistungsqualität) -> Dienstleistungsqualität: 0/1, Mux4/2
  Güterangebotsqualität: 0/1 -> Populationsmodell/3(Güterangebotsqualität bei vorhandem Einkommen)
  "Arbeitsplätze Unternehmen: 10 "/1 -> Mux9/5, Mux7/4, Haushalte/7(Arbeitsplätze Unternehmen)
  Kreditrückzahlung: 0/1 -> Mux9/6, Haushalte/8(Kreditrückzahlung Ausland)
  Neue Kreditvergabe: 0/1 -> Mux9/4, Haushalte/6(Neue Kreditvergabe Inland)
  Arbeitslohn: 4/1 -> Mux8/1, Haushalte/4(Arbeitslohn), Mux7/2, Mux4/4, Öffentliche Dienstleistungen/3(Arbeitslohn)
  Güterangebot: 0/1 -> Mux7/3, Mux9/3, Haushalte/3(Güterangebot Inland), Scope5/1
  Arbeitsplätze Unternehmen: 5/1 -> Haushalte/2(Arbeitsplätze Dienstleistungen), Mux9/2
  Erwerbstätige: 30/1 -> Haushalte/1(Erwerbsfähige), Mux9/1
  Güterkonsum: 50/1 -> Unternehmen/5(Güterkonsum Inland), Mux11/1
  Mux4/1 -> Scope9/1
  Staat/3(Geldbestand Staat) -> Mux2/3
  Mux2/1 -> Scope2/1
  Mux5/1 -> Scope2/2
  Mux/1 -> Bank/1
  Mux7/1 -> Scope10/1
  Mux1/1 -> Bank/2
  Mux6/1 -> "Haushalte "/1
  Mux8/1 -> "Haushalte "/3
  Haushalte/6(Gütervorrat der Haushalte) -> Mux6/6
  Mux9/1 -> "Haushalte "/2
  Mux3/1 -> "Unternehmen "/1
  Mux10/1 -> "Unternehmen "/2
  Mux11/1 -> "Unternehmen "/3
  Güterkonsum Ausland/1 -> Güterkonsum Ausland: 0/1
  Zinssatz Ausland: 0.03/1 -> Haushalte/14(Kreditzinssatz Ausland), Unternehmen/9(Kreditzinssatz Ausland)
  Unternehmen/15(Güterangebot Ausland) -> Güterangebot an  Ausland/1
  Kreditbedarf Haushalte: 0/1 -> Banken/2(Kreditbedarf der Haushalte)
  Kreditbedarf Unternehmen: 0/1 -> Banken/3(Kreditbedarf der Unternehmen)
  Einlagenänderung Haushalte: 0/1 -> Banken/1(Einlangenänderung der Haushalte)
  Kreditbedarf der Haushalte im Ausland: 0/1 -> Banken/4(Kreditbedarf der Haushalte im Ausland)
  Kreditbedarf der Unternehmen im Ausland: 0/1 -> Banken/5(Kreditbedarf der Unternehmen im Ausland)
  Neue Kreditvergabe der Unternehmen Ausland/1 -> Neue Kreditvergabe der Unternehmen Ausland: 0/1
  Kreditrückzahlung der Unternehmen Ausland/1 -> Kreditrückzahlung der Unternehmen Ausland: 0/1
  Banken/16(Kreditrückzahlung der Unternehmen im Ausland) -> Bank: Kreditrückzahlung der Unternemen Ausland/1
  Banken/18(Kredite der Haushalte im Ausland) -> Kredite gesammt/5
  Banken/15(Kredite der Unternehmen im Ausland) -> Kredite gesammt/4
  Neue Kreditvergabe der Haushalte Ausland/1 -> Neue Kreditvergabe der Haushalte Ausland: 0/1
  Unternehmen/11(Kreditbedarf Ausland) -> Kreditbedarf Ausland Unternehmen/1
  Kreditrückzahlung der Haushalte Ausland/1 -> Kreditrückzahlung der Haushalte Ausland: 0/1
  Haushalte/10(Kreditbedarf Ausland) -> Kreditbedarf Ausland Haushalte/1
  Banken/20(Kreditvergabe der Haushalte im Ausland) -> "Bank: Kreditvergabe der Haushalte Ausland "/1
  Güterangebot vom  Ausland/1 -> Güterangebot vom  Ausland: 0/1
  Unternehmen/6(zukünftiger Arbeitsdarf der Unternehmen) -> zukünftiger Arbeitsdebdarf/1
  Banken/17(Kreditvergabe der Unternehmen im Ausland) -> "Bank: Kreditvergabe der Unternemen Ausland "/1
  Banken/19(Kreditrückzahlung der Haushalte im Ausland) -> Bank: Kreditrückzahlung der Haushalte Ausland/1
  Güterpreis: 3/1 -> Güterpreis/1, Mux7/1, Mux8/2, Haushalte/5(Güterpreis Inland)
  Kreditbedarf der Haushalte im Ausland/1 -> Kreditbedarf der Haushalte im Ausland: 0/1
  Kreditbedarf der Unternehmen im Ausland/1 -> Kreditbedarf der Unternehmen im Ausland: 0/1
  Güterkonsum Ausland: 0/1 -> Mux13/7, Wechselkursberechnung/3(Güterkonsum im Ausland von Gütern im Inland), Unternehmen/6(Güterkonsum Ausland)
  Zinssatz Ausland/1 -> Zinssatz Ausland: 0.03/1
  Neue Kreditvergabe der Unternehmen Ausland: 0/1 -> Unternehmen/11(Neue Kreditvergabe der Unternehmen Ausland)
  Kreditrückzahlung der Unternehmen Ausland: 0/1 -> Unternehmen/12(Kreditrückzahlung der Unternehmen Ausland)
  Güterpreis Ausland: 5/1 -> Mux13/5, Wechselkursberechnung/1(Güterpreis Ausland)
  Neue Kreditvergabe der Haushalte Ausland: 0/1 -> Haushalte/10(Neue Kreditvergabe Ausland)
  Kreditrückzahlung der Haushalte Ausland: 0/1 -> Haushalte/11(Kreditrückzahlung Inland)
  Güterangebot vom  Ausland: 0/1 -> Haushalte/12(Güterangebot Ausland)
  Mux14/1 -> Bank1/1
  Mux12/1 -> Bank1/2
  Arbeitslosenquote: 0/1 -> Notenbank/2(Arbeitslosenquote), Mux12/1
  Güterpreis Ausland/1 -> Güterpreis Ausland: 5/1
  Wechselkursberechnung/1(Güterpreis Ausland in Eigenwährung) -> Güterpreis Ausland in Eigenwährung: 4/1, Mux13/1
  Haushalte/9(Güterkonsum Ausland) -> Mux13/6, Wechselkursberechnung/2(Güterkonsum im Inland von Gütern vom Ausland), Güterkonsum vom Ausland/1
  Güterpreis Ausland in Eigenwährung: 4/1 -> Haushalte/9(Güterpreis Ausland)
  Wechselkursberechnung/3(Gesamter Güterkonsum im Ausland von Gütern im Inland) -> Mux13/3
  Wechselkursberechnung/2(Wechselkursfaktor) -> Mux13/2
  Wechselkursberechnung/4(Gesamter Güterkonsum im Inland von Gütern vom Ausland) -> Mux13/4
  Mux13/1 -> Wechselkurszustände/1
